simulink model "bus_selector1"  (Simulink 4.00)
settings: Solver=ode45  StartTime=0.0  StopTime=10.0  RelTol=1e-3
libraries: simulink3 x1
settings Model: LastModifiedBy=Administrator  Refine=5  BlockReductionOpt=off

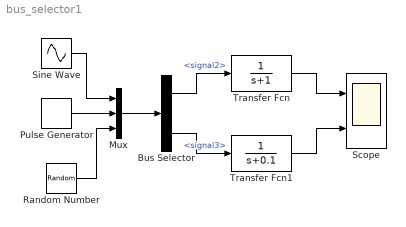
== system bus_selector1 ==
  Bus Selector : BusSelector  OutputSignals=signal2,signal3  MuxedOutput=off
  Mux : Mux  Inputs=3
  Pulse Generator : simulink3/Sources/Pulse Generator  period=1  duty=50  amplitude=1  start=0
  Random Number : RandomNumber  Mean=0  Variance=1  Seed=0  SampleTime=0
  Scope : Scope  NumInputPorts=2
      settings: TimeRange=auto  YMin=-5~-5  YMax=5~5  SaveToWorkspace=off  SaveName=ScopeData  LimitDataPoints=on  MaxDataPoints=5000
  Sine Wave : Sin  Amplitude=1  Frequency=1  Phase=0  SampleTime=0
  Transfer Fcn : TransferFcn  Numerator=[1]  Denominator=[1 1]  Realization=auto  AbsoluteTolerance=auto
  Transfer Fcn1 : TransferFcn  Numerator=[1]  Denominator=[1 0.1]  Realization=auto  AbsoluteTolerance=auto
  wires:
  Mux/1 -> Bus Selector/1
  Sine Wave/1 -> Mux/1
  Pulse Generator/1 -> Mux/2
  Transfer Fcn1/1 -> Scope/2
  Transfer Fcn/1 -> Scope/1
  Bus Selector/1 -> Transfer Fcn/1  "<signal2>"
  Bus Selector/2 -> Transfer Fcn1/1  "<signal3>"
  Random Number/1 -> Mux/3
